simulink library "csu_tss_thrustersim_sim_lib"  (R2014b)
settings: Solver=ode45  StartTime=0.0  StopTime=10.0  RelTol=1e-3
libraries: simulink x2, util_info_lib x1
settings Model: Creator=escrane  LastModifiedBy=mstewart

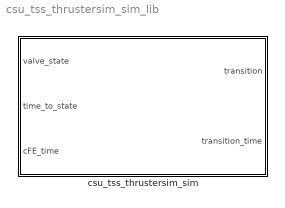
== system csu_tss_thrustersim_sim_lib ==
  csu_tss_thrustersim_sim : Subsystem

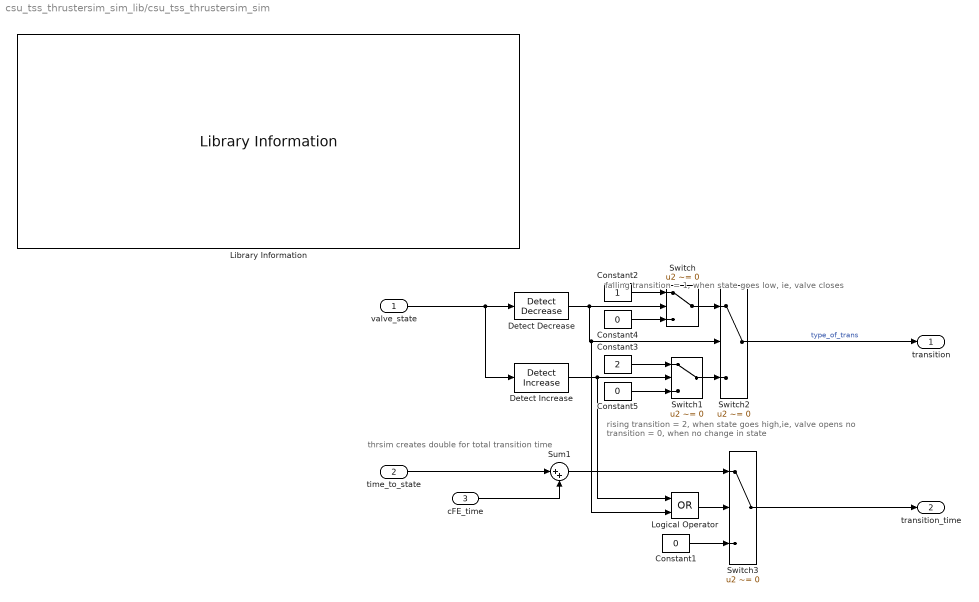
== system csu_tss_thrustersim_sim_lib/csu_tss_thrustersim_sim ==
  note: falling transition = 1, when state goes low, ie, valve closes
  note: rising transition = 2, when state goes high,ie, valve opens
      | no transition = 0, when no change in state
  note: thrsim creates double for total transition time
  valve_state : Inport
  time_to_state : Inport  Port=2
  cFE_time : Inport  Port=3
  Constant1 : Constant  Value=0  OutDataTypeStr=double
  Constant2 : Constant  OutDataTypeStr=uint8
  Constant3 : Constant  Value=2  OutDataTypeStr=uint8
  Constant4 : Constant  Value=0  OutDataTypeStr=uint8
  Constant5 : Constant  Value=0  OutDataTypeStr=uint8
  Detect Decrease : simulink/Logic and Bit Operations/Detect Decrease  vinit=0.0  InputProcessing=Inherited  OutDataTypeStr=uint8
  Detect Increase : simulink/Logic and Bit Operations/Detect Increase  vinit=0.0  InputProcessing=Inherited  OutDataTypeStr=uint8
  Library Information : util_info_lib/Library Information  owner='escrane'
  Logical Operator : Logic  Operator=OR  AllPortsSameDT=off  OutDataTypeStr=boolean
  Sum1 : Sum  Inputs=|++
  Switch{,1..3} (4 alike) : Switch  Criteria=u2 ~= 0
  transition : Outport
  transition_time : Outport  Port=2
  wires:
  Constant1/1 -> Switch3/3
  Detect Increase/1 -> Switch1/2, Logical Operator/1
  Logical Operator/1 -> Switch3/2
  Switch3/1 -> transition_time/1
  Sum1/1 -> Switch3/1
  Switch2/1 -> transition/1  "type_of_trans"
  valve_state/1 -> Detect Increase/1, Detect Decrease/1
  Detect Decrease/1 -> Switch2/2, Logical Operator/2, Switch/2
  Constant2/1 -> Switch/1
  Constant3/1 -> Switch1/1
  Constant4/1 -> Switch/3
  Constant5/1 -> Switch1/3
  Switch/1 -> Switch2/1
  Switch1/1 -> Switch2/3
  time_to_state/1 -> Sum1/1
  cFE_time/1 -> Sum1/2
